simulink model "Throttle_harness"  (Simulink 7.7)
settings: Solver=FixedStepDiscrete  SolverMode=SingleTasking  StartTime=0.0  StopTime=100  FixedStep=.01  RelTol=1e-3
InitFcn:
  | if signalbuilder('Throttle_harness/Signal_Builder','activegroup') == 1
  |    CD_THROTTLE_PRIMARY_FUNCTION.DataType = 'uint8';
  |    CD_THROTTLE_PRIMARY_FUNCTION.Value = 255;
  | else
  |    CD_THROTTLE_PRIMARY_FUNCTION.DataType = 'uint8';
  |    CD_THROTTLE_PRIMARY_FUNCTION.Value = 0;
  | end
  | 
  | 
  | if signalbuilder('Throttle_harness/Signal_Builder','activegroup') == 3
  |    CD_THROTTLE_PRIMARY_DEBOUNCE_NORMAL.DataType = 'uint16';
  |    CD_THROTTLE_PRIMARY_DEBOUNCE_NORMAL.Value = 65535;
  | else
  |    CD_THROTTLE_PRIMARY_DEBOUNCE_NORMAL.DataType = 'uint16';
  |    CD_THROTTLE_PRIMARY_DEBOUNCE_NORMAL.Value = 10;
  | end
undefined symbols (not defined in the file): ACTIVE, CD_THROTTLE_FAULT_DERATE, CD_THROTTLE_PRI_RATIO_HIGH, CD_THROTTLE_PRI_RATIO_LOW, CD_THROTTLE_PRIMARY_DEBOUNCE_OORH, CD_THROTTLE_PRIMARY_DEBOUNCE_OORL, CD_THROTTLE_PRIMARY_FILTER_GAIN, CD_THROTTLE_PRIMARY_OORH, CD_THROTTLE_PRIMARY_OORL, INACTIVE, NON_FUNCTIONAL, NORMAL, OORH, OORL, sigbuilder_block, srate100, UNLIMITED
libraries: MX_Library x4, simulink x1
CloseFcn:
  | rtwprivate ssgencode ModelCloseRequest sle_main_controller
settings Model: Creator=spencermindeman  LastModifiedBy=aliebel  CovMetricSettings=dcmw  CovHTMLOptions=-aTS=1 -bRG=1 -bTC=1 -hTR=0 -nFC=0 -scm=1 -bcm=1 -xEv=0  covSaveCumulativeToWorkspaceVar=off  CovSaveSingleToWorkspaceVar=off  CovModelRefEnable=off
settings MATStruct: SampleTime=0.01  Offset=0  Priority=[1.0]
settings DataIOCC: LimitDataPoints=off  SaveOutput=off  SaveTime=off
settings OptimizationCC: BlockReduction=off  InlineParams=on  ExpressionFolding=off  StateBitsets=on  DataBitsets=on  UseTempVars=on  InitFltsAndDblsToZero=on  NoFixptDivByZeroProtection=on  EfficientFloat2IntCast=on  OptimizeModelRefInitCode=on
settings DebuggingCC: SaveWithParameterizedLinksMsg=none  MultiTaskDSMMsg=warning  MultiTaskCondExecSysMsg=none  IntegerOverflowMsg=none  ModelReferenceCSMismatchMessage=warning
settings HardwareCC: ProdBitPerInt=16  ProdBitPerPointer=16  ProdIntDivRoundTo=Floor  ProdEndianess=BigEndian  ProdWordSize=16  ProdHWDeviceType=Motorola HC12
settings ModelReferenceCC: ModelReferenceNumInstancesAllowed=Single
settings RTWCC: SystemTargetFile=ert.tlc  GenCodeOnly=on  TemplateMakefile=ert_default_tmf  Description=Real-Time Workshop Embedded Coder (no auto configuration)  GenerateReport=on  RetainRTWFile=on  ProcessScript=ert_make_rtw_hook  IncludeHyperlinkInReport=on  LaunchReport=on  IncludeERTFirstTime=on
settings RTWCC: CustomHeaderCode=|
  | #include "cpp_req_defines.h"
  | #include "hw_fin.h"
  | #include "cdata.h"
settings CodeAppCC: IgnoreCustomStorageClasses=off  DefineNamingRule=UpperCase
settings ERTTargetCC: TargetFcnLib=ansi_tfl_tmw.mat  FunctionExecutionProfile=off  MultiwordLength=2048  GenerateSampleERTMain=on  IncludeMdlTerminateFcn=off  SupportAbsoluteTime=off  SupportNonFinite=off  SupportComplex=off  PurelyIntegerCode=on  ERTCustomFileTemplate=gen_rtw_req_defines_h.tlc  GlobalDataDefinition=InSeparateSourceFile  GlobalDataReference=InSeparateHeaderFile  ConvertIfToSwitch=off

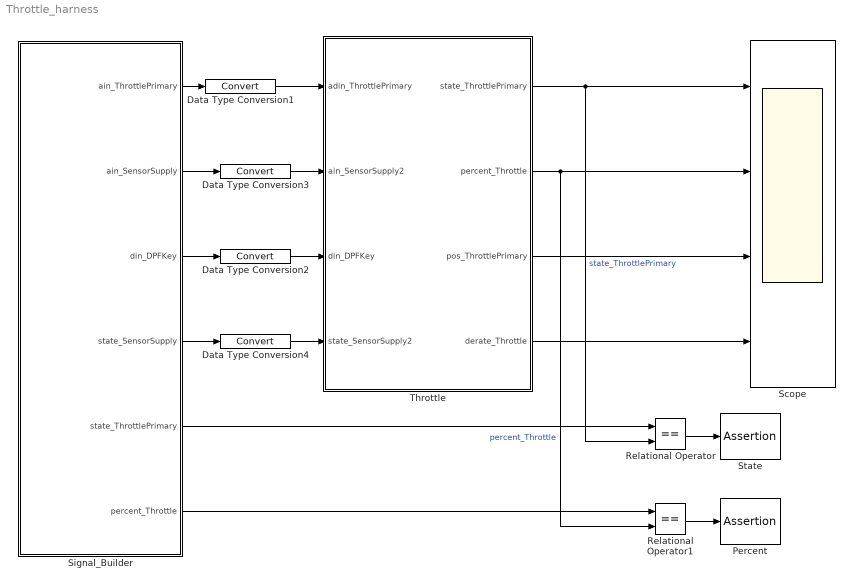
== system Throttle_harness ==
  Data Type Conversion{1..4} (4 alike) : DataTypeConversion
  Percent : Assertion  Enabled=off
  Relational Operator : RelationalOperator  Operator===  OutDataTypeStr=boolean
  Relational Operator1 : RelationalOperator  Operator===  OutDataTypeStr=boolean
  Scope : Scope  NumInputPorts=4
      settings: TimeRange=100  YMin=7.5~7.5~60~0  YMax=22.5~22.5~120~300  MaxDataPoints=50000
  Signal_Builder : Subsystem  Tag=STV Subsys  LoadFcn=sigbuilder_block('load');  StartFcn=sigbuilder_block('start');  StopFcn=sigbuilder_block('stop');  ClipboardFcn=sigbuilder_block('clipboard');  mask(Sigbuilder block){}
      mask help: Sigbuilder GUI
      mask init:
      | if ~strcmp(get_param(bdroot(gcbh),'SimulationStatus'),'stopped') tuvar = sigbuilder_block('maskInit'); end
      settings: CopyFcn=sigbuilder_block('copy');  DeleteFcn=sigbuilder_block('delete');  ModelCloseFcn=sigbuilder_block('modelClose');  PreSaveFcn=sigbuilder_block('preSave');  NameChangeFcn=sigbuilder_block('namechange');  OpenFcn=sigbuilder_block('open',[456.75 122.25 954 619.5 ]);  CloseFcn=sigbuilder_block('close');
      mask Display: plot(0,0,100,100,[10,10,40,40,10],[80,20,20,80,80],[40,10],[50,50], [40,27,10],[65,72,56],[40,25,25,10],[28,28,43,43]);
  State : Assertion  Enabled=off
  Throttle : Subsystem  TreatAsAtomicUnit=on  SystemSampleTime=srate100  RTWFileName=mod_Inputs
      settings: RTWSystemCode=Function  RTWFileNameOpts=User specified
  wires:
  Relational Operator/1 -> State/1
  Signal_Builder/1(ain_ThrottlePrimary) -> Data Type Conversion1/1
  Signal_Builder/3(din_DPFKey) -> Data Type Conversion2/1
  Data Type Conversion1/1 -> Throttle/1(adin_ThrottlePrimary)
  Data Type Conversion2/1 -> Throttle/3(din_DPFKey)
  Data Type Conversion3/1 -> Throttle/2(ain_SensorSupply2)
  Data Type Conversion4/1 -> Throttle/4(state_SensorSupply2)
  Throttle/1(state_ThrottlePrimary) -> Scope/1, Relational Operator/2  "state_ThrottlePrimary"
  Signal_Builder/2(ain_SensorSupply) -> Data Type Conversion3/1
  Signal_Builder/4(state_SensorSupply) -> Data Type Conversion4/1
  Signal_Builder/5(state_ThrottlePrimary) -> Relational Operator/1
  Relational Operator1/1 -> Percent/1
  Signal_Builder/6(percent_Throttle) -> Relational Operator1/1
  Throttle/2(percent_Throttle) -> Scope/2, Relational Operator1/2  "percent_Throttle"
  Throttle/3(pos_ThrottlePrimary) -> Scope/3
  Throttle/4(derate_Throttle) -> Scope/4

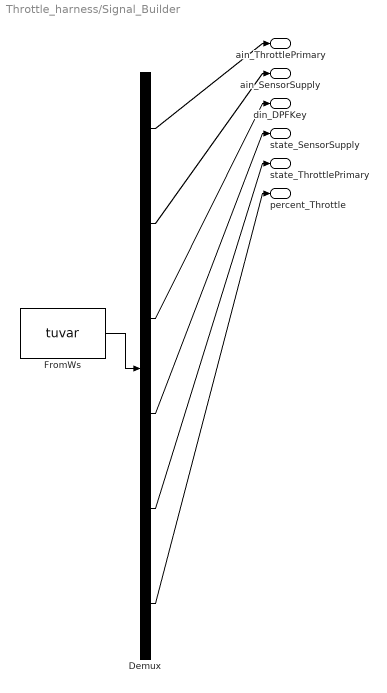
== system Throttle_harness/Signal_Builder ==
  Demux : Demux  Tag=STV Demux  Outputs=6
  FromWs : FromWorkspace  Tag=STV FromWs  VariableName=tuvar  SampleTime=0  SigBuilderData=DataTag0  VnvData=DataTag1
      SigBuilderData=|
      | common.afterFinalStr = 'Extrapolate'
      | common.sampleTime = 0
      | dataSet(1).timeRange = [0 100]
      | dataSet(1).name = 'T1-nonfunc'
      | dataSet(2).timeRange = [0 100]
      | dataSet(2).name = 'T2-OOR'
      | dataSet(3).timeRange = [0 100]
      | dataSet(3).name = 'T3-OOR_UNLIMITED'
      | dataSet(4).timeRange = [0 100]
      | dataSet(4).name = 'T4-Primary Only'
      | dataSet(5).timeRange = [0 100]
      | dataSet(5).name = 'T5-DPF Key'
      | sbobj.Groups(1).Name = 'T1-nonfunc'
      | sbobj.Groups(1).Signals(1).Name = 'ain_ThrottlePrimary'
      | sbobj.Groups(1).Signals(1).XData = [0 50 100]
      | sbobj.Groups(1).Signals(1).YData = [17 83 17]
      | sbobj.Groups(1).Signals(2).Name = 'ain_SensorSupply'
      | sbobj.Groups(1).Signals(2).XData = [0 100]
      | sbobj.Groups(1).Signals(2).YData = [500 500]
      | sbobj.Groups(1).Signals(3).Name = 'din_DPFKey'
      | sbobj.Groups(1).Signals(3).XData = [0 100]
      | sbobj.Groups(1).Signals(3).YData = [0 0]
      | sbobj.Groups(1).Signals(4).Name = 'state_SensorSupply'
      | sbobj.Groups(1).Signals(4).XData = [0 100]
      | sbobj.Groups(1).Signals(4).YData = [8 8]
      | sbobj.Groups(1).Signals(5).Name = 'state_ThrottlePrimary'
      | sbobj.Groups(1).Signals(5).XData = [0 100]
      | sbobj.Groups(1).Signals(5).YData = [8 8]
      | sbobj.Groups(1).Signals(6).Name = 'percent_Throttle'
      | sbobj.Groups(1).Signals(6).XData = [0 100]
      | sbobj.Groups(1).Signals(6).YData = [0 0]
      | sbobj.Groups(2).Name = 'T2-OOR'
      | sbobj.Groups(2).Signals(1).Name = 'ain_ThrottlePrimary'
      | sbobj.Groups(2).Signals(1).XData = [0 6.5 6.5 7.6 7.6 9.9 9.9 20 20 20.5 20.5 24.5 24.5 30 30 30.5 30.5 33.7 33.7 38.2 38.2 39.1 39.1 40 40 52.2 52.2 53.9 53.9 62.9 62.9 65.2 65.2 72 72 78 78 82.8 82.8 86.1 86.1 92.1 92.1 94.4 94.4 100]
      | sbobj.Groups(2).Signals(1).YData = [25 25 0 0 25 25 0 0 25 25 0 0 25 25 1023 1023 25 25 1023 1023 25 25 1023 1023 25 25 1023 1023 25 25 0 0 25 25 1023 1023 25 25 0 0 25 25 0 0 1023 1023]
      | sbobj.Groups(2).Signals(2).Name = 'ain_SensorSupply'
      | sbobj.Groups(2).Signals(2).XData = [0 100]
      | sbobj.Groups(2).Signals(2).YData = [500 500]
      | sbobj.Groups(2).Signals(3).Name = 'din_DPFKey'
      | sbobj.Groups(2).Signals(3).XData = [0 100]
      | sbobj.Groups(2).Signals(3).YData = [0 0]
      | sbobj.Groups(2).Signals(4).Name = 'state_SensorSupply'
      | sbobj.Groups(2).Signals(4).XData = [0 52.2 52.2 54.4 54.4 61.6 61.6 65.4 65.4 73.2 73.2 80.1 80.1 84.8 84.8 89.6 89.6 100]
      | sbobj.Groups(2).Signals(4).YData = [8 8 22 22 8 8 21 21 8 8 22 22 8 8 21 21 8 8]
      | sbobj.Groups(2).Signals(5).Name = 'state_ThrottlePrimary'
      | sbobj.Groups(2).Signals(5).XData = [0 11.8 11.8 25.8 25.8 35.2 35.2 41.5 41.5 84.8 84.8 87.4 87.4 94 94 95.9 95.9 100]
      | sbobj.Groups(2).Signals(5).YData = [8 8 22 22 8 8 21 21 8 8 22 22 8 8 22 22 21 21]
      | sbobj.Groups(2).Signals(6).Name = 'percent_Throttle'
      | sbobj.Groups(2).Signals(6).XData = [0 0.1 0.1 11.8 11.8 25.9 25.9 35.2 35.2 41.6 41.6 52.2 52.2 54.6 54.6 61.6 61.6 65.5 65.5 73.2 73.2 80.2 80.2 84.8 84.8 89.7 89.7 94 94 100]
      | sbobj.Groups(2).Signals(6).YData = [0 0 46 46 500 500 46 46 500 500 46 46 500 500 46 46 500 500 46 46 500 500 46 46 500 500 46 46 500 500]
      | sbobj.Groups(3).Name = 'T3-OOR_UNLIMITED'
      | sbobj.Groups(3).Signals(1).Name = 'ain_ThrottlePrimary'
      | sbobj.Groups(3).Signals(1).XData = [0 6.5 6.5 7.6 7.6 9.9 9.9 20 20 20.5 20.5 24.5 24.5 30 30 30.5 30.5 33.7 33.7 38.2 38.2 39.1 39.1 40 40 100]
      | sbobj.Groups(3).Signals(1).YData = [25 25 0 0 25 25 0 0 25 25 0 0 25 25 1023 1023 25 25 1023 1023 25 25 1023 1023 25 25]
      | sbobj.Groups(3).Signals(2).Name = 'ain_SensorSupply'
      | sbobj.Groups(3).Signals(2).XData = [0 100]
      | sbobj.Groups(3).Signals(2).YData = [500 500]
      | sbobj.Groups(3).Signals(3).Name = 'din_DPFKey'
      | sbobj.Groups(3).Signals(3).XData = [0 100]
      | sbobj.Groups(3).Signals(3).YData = [0 0]
      | sbobj.Groups(3).Signals(4).Name = 'state_SensorSupply'
      | sbobj.Groups(3).Signals(4).XData = [0 100]
      | sbobj.Groups(3).Signals(4).YData = [8 8]
      | sbobj.Groups(3).Signals(5).Name = 'state_ThrottlePrimary'
      | sbobj.Groups(3).Signals(5).XData = [0 11.8 11.8 35.2 35.2 100]
      | sbobj.Groups(3).Signals(5).YData = [8 8 22 22 21 21]
      | sbobj.Groups(3).Signals(6).Name = 'percent_Throttle'
      | sbobj.Groups(3).Signals(6).XData = [0 0.1 0.1 11.8 11.8 100]
      | sbobj.Groups(3).Signals(6).YData = [0 0 46 46 500 500]
      | sbobj.Groups(4).Name = 'T4-Primary Only'
      | sbobj.Groups(4).Signals(1).Name = 'ain_ThrottlePrimary'
      | sbobj.Groups(4).Signals(1).XData = [0 30 30 40 40 100]
      | sbobj.Groups(4).Signals(1).YData = [25 25 0 0 25 25]
      | sbobj.Groups(4).Signals(2).Name = 'ain_SensorSupply'
      | sbobj.Groups(4).Signals(2).XData = [0 100]
      | sbobj.Groups(4).Signals(2).YData = [500 500]
      | sbobj.Groups(4).Signals(3).Name = 'din_DPFKey'
      | sbobj.Groups(4).Signals(3).XData = [0 100]
      | sbobj.Groups(4).Signals(3).YData = [0 0]
      | sbobj.Groups(4).Signals(4).Name = 'state_SensorSupply'
      | sbobj.Groups(4).Signals(4).XData = [0 10 10 20 20 100]
      | sbobj.Groups(4).Signals(4).YData = [8 8 21 21 8 8]
      | sbobj.Groups(4).Signals(5).Name = 'state_ThrottlePrimary'
      | sbobj.Groups(4).Signals(5).XData = [0 31.9 31.9 41.3 41.3 100]
      | sbobj.Groups(4).Signals(5).YData = [8 8 22 22 8 8]
      | sbobj.Groups(4).Signals(6).Name = 'percent_Throttle'
      | sbobj.Groups(4).Signals(6).XData = [0 0.1 0.1 10 10 20.1 20.1 31.9 31.9 41.4 41.4 100]
      | sbobj.Groups(4).Signals(6).YData = [0 0 46 46 500 500 46 46 500 500 46 46]
      | sbobj.Groups(5).Name = 'T5-DPF Key'
      | sbobj.Groups(5).Signals(1).Name = 'ain_ThrottlePrimary'
      | sbobj.Groups(5).Signals(1).XData = [0 20 30 59.9 74.8 100]
      | sbobj.Groups(5).Signals(1).YData = [25 25 25 25 25 25]
      | sbobj.Groups(5).Signals(2).Name = 'ain_SensorSupply'
      | sbobj.Groups(5).Signals(2).XData = [0 100]
      | sbobj.Groups(5).Signals(2).YData = [500 500]
      | sbobj.Groups(5).Signals(3).Name = 'din_DPFKey'
      | sbobj.Groups(5).Signals(3).XData = [0 5.4 5.4 7.2 7.2 18.8 18.8 20.3 20.3 100]
      | sbobj.Groups(5).Signals(3).YData = [0 0 1 1 0 0 1 1 0 0]
      | sbobj.Groups(5).Signals(4).Name = 'state_SensorSupply'
      | sbobj.Groups(5).Signals(4).XData = [0 17.4 17.4 21.4 21.4 100]
      | sbobj.Groups(5).Signals(4).YData = [8 8 21 21 8 8]
      | sbobj.Groups(5).Signals(5).Name = 'state_ThrottlePrimary'
      | sbobj.Groups(5).Signals(5).XData = [0 100]
      | sbobj.Groups(5).Signals(5).YData = [8 8]
      | sbobj.Groups(5).Signals(6).Name = 'percent_Throttle'
      | sbobj.Groups(5).Signals(6).XData = [0 0.1 0.1 5.4 5.4 7.3 7.3 17.4 17.4 18.8 18.8 20.4 20.4 21.5 21.5 100]
      | sbobj.Groups(5).Signals(6).YData = [0 0 46 46 0 0 46 46 500 500 0 0 500 500 46 46]
  ain_ThrottlePrimary : Outport  Tag=STV Outport
  ain_SensorSupply : Outport  Tag=STV Outport  Port=2
  din_DPFKey : Outport  Tag=STV Outport  Port=3
  state_SensorSupply : Outport  Tag=STV Outport  Port=4
  state_ThrottlePrimary : Outport  Tag=STV Outport  Port=5
  percent_Throttle : Outport  Tag=STV Outport  Port=6
  wires:
  FromWs/1 -> Demux/1
  Demux/1 -> ain_ThrottlePrimary/1
  Demux/2 -> ain_SensorSupply/1
  Demux/3 -> din_DPFKey/1
  Demux/4 -> state_SensorSupply/1
  Demux/5 -> state_ThrottlePrimary/1
  Demux/6 -> percent_Throttle/1

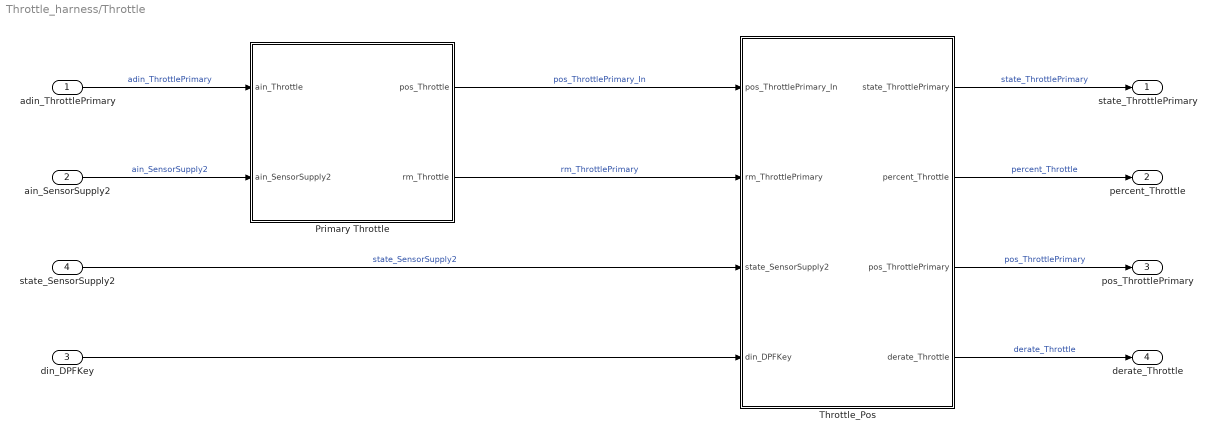
== system Throttle_harness/Throttle ==
  adin_ThrottlePrimary : Inport  OutDataTypeStr=uint16
  ain_SensorSupply2 : Inport  Port=2  OutDataTypeStr=uint16
  din_DPFKey : Inport  Port=3
  state_SensorSupply2 : Inport  Port=4  OutDataTypeStr=uint8
  Primary Throttle : Subsystem
  Throttle_Pos : Stateflow chart  TreatAsAtomicUnit=on
  state_ThrottlePrimary : Outport
  percent_Throttle : Outport  Port=2
  pos_ThrottlePrimary : Outport  Port=3
  derate_Throttle : Outport  Port=4
  wires:
  adin_ThrottlePrimary/1 -> Primary Throttle/1(ain_Throttle)  "adin_ThrottlePrimary"
  Throttle_Pos/1(state_ThrottlePrimary) -> state_ThrottlePrimary/1  "state_ThrottlePrimary"
  ain_SensorSupply2/1 -> Primary Throttle/2(ain_SensorSupply2)  "ain_SensorSupply2"
  Throttle_Pos/2(percent_Throttle) -> percent_Throttle/1  "percent_Throttle"
  Primary Throttle/1(pos_Throttle) -> Throttle_Pos/1(pos_ThrottlePrimary_In)  "pos_ThrottlePrimary_In"
  Primary Throttle/2(rm_Throttle) -> Throttle_Pos/2(rm_ThrottlePrimary)  "rm_ThrottlePrimary"
  Throttle_Pos/3(pos_ThrottlePrimary) -> pos_ThrottlePrimary/1  "pos_ThrottlePrimary"
  state_SensorSupply2/1 -> Throttle_Pos/3(state_SensorSupply2)  "state_SensorSupply2"
  Throttle_Pos/4(derate_Throttle) -> derate_Throttle/1  "derate_Throttle"
  din_DPFKey/1 -> Throttle_Pos/4(din_DPFKey)

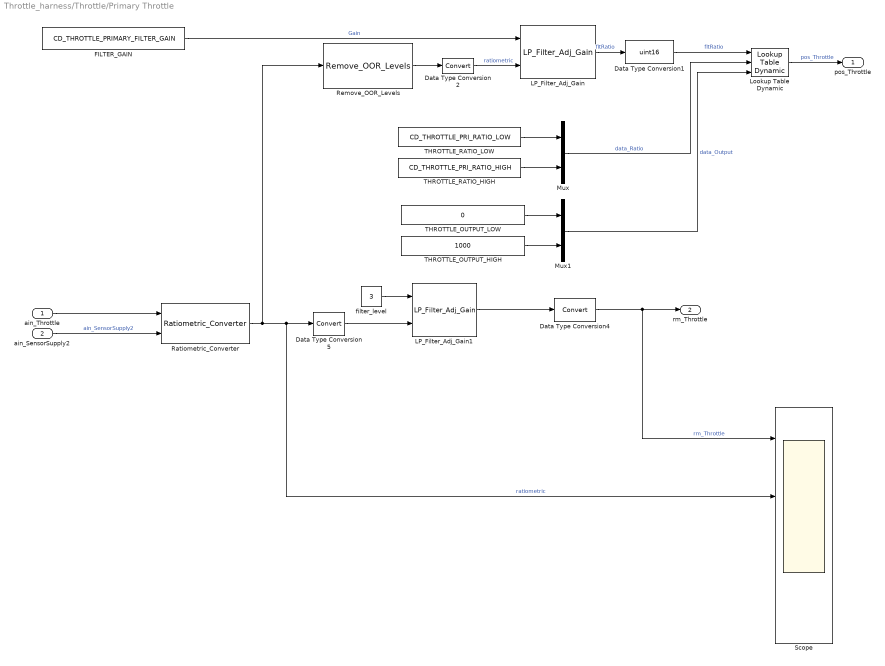
== system Throttle_harness/Throttle/Primary Throttle ==
  ain_Throttle : Inport
  ain_SensorSupply2 : Inport  Port=2
  Data Type Conversion1 : DataTypeConversion  OutDataTypeStr=uint16
  Data Type Conversion2 : DataTypeConversion
  Data Type Conversion4 : DataTypeConversion
  Data Type Conversion5 : DataTypeConversion
  FILTER_GAIN : Constant  Value=CD_THROTTLE_PRIMARY_FILTER_GAIN  OutDataTypeStr=uint8  SampleTime=-1
  LP_Filter_Adj_Gain : MX_Library/LP_Filter_Adj_Gain  SystemSampleTime=-1
  LP_Filter_Adj_Gain1 : MX_Library/LP_Filter_Adj_Gain  SystemSampleTime=-1
  Lookup Table Dynamic : simulink/Lookup Tables/Lookup Table Dynamic  LookUpMeth=Interpolation-Use End Values  OutDataTypeStr=fixdt(0,16,0)  OutputDataTypeScalingMode=Specify via dialog  OutDataType=fixdt(0,16,0)  OutScaling=[]  DoSatur=off
  Mux : Mux  Inputs=2
  Mux1 : Mux  Inputs=2
  Ratiometric_Converter : MX_Library/Ratiometric_Converter  SystemSampleTime=-1  multiplier=CD_THROTTLE_PRIMARY_RATIO_MULTIPLIER
  Remove_OOR_Levels : MX_Library/Remove_OOR_Levels  SystemSampleTime=-1  OORL_LEVEL=50  OORH_LEVEL=950
  Scope : Scope  NumInputPorts=4
      settings: TimeRange=100  YMin=7.5~7.5~60~0  YMax=22.5~22.5~120~300  MaxDataPoints=50000
  THROTTLE_OUTPUT_HIGH : Constant  Value=1000  OutDataTypeStr=uint16  SampleTime=-1
  THROTTLE_OUTPUT_LOW : Constant  Value=0  OutDataTypeStr=uint16  SampleTime=-1
  THROTTLE_RATIO_HIGH : Constant  Value=CD_THROTTLE_PRI_RATIO_HIGH  OutDataTypeStr=uint16  SampleTime=-1
  THROTTLE_RATIO_LOW : Constant  Value=CD_THROTTLE_PRI_RATIO_LOW  OutDataTypeStr=uint16  SampleTime=-1
  filter_level : Constant  Value=3  OutDataTypeStr=uint8  SampleTime=-1
  pos_Throttle : Outport
  rm_Throttle : Outport  Port=2
  wires:
  Data Type Conversion5/1 -> LP_Filter_Adj_Gain1/2
  filter_level/1 -> LP_Filter_Adj_Gain1/1
  LP_Filter_Adj_Gain1/1 -> Data Type Conversion4/1
  Data Type Conversion2/1 -> LP_Filter_Adj_Gain/2  "ratiometric"
  Remove_OOR_Levels/1 -> Data Type Conversion2/1
  Data Type Conversion4/1 -> rm_Throttle/1, Scope/1  "rm_Throttle"
  Ratiometric_Converter/1 -> Remove_OOR_Levels/1, Data Type Conversion5/1, Scope/2  "ratiometric"
  FILTER_GAIN/1 -> LP_Filter_Adj_Gain/1  "Gain"
  Data Type Conversion1/1 -> Lookup Table Dynamic/1  "fltRatio"
  LP_Filter_Adj_Gain/1 -> Data Type Conversion1/1  "fltRatio"
  ain_SensorSupply2/1 -> Ratiometric_Converter/2  "ain_SensorSupply2"
  ain_Throttle/1 -> Ratiometric_Converter/1
  Lookup Table Dynamic/1 -> pos_Throttle/1  "pos_Throttle"
  THROTTLE_RATIO_LOW/1 -> Mux/1
  THROTTLE_OUTPUT_HIGH/1 -> Mux1/2
  Mux/1 -> Lookup Table Dynamic/2  "data_Ratio"
  THROTTLE_OUTPUT_LOW/1 -> Mux1/1
  Mux1/1 -> Lookup Table Dynamic/3  "data_Output"
  THROTTLE_RATIO_HIGH/1 -> Mux/2

== stateflow chart Throttle/Throttle_Pos ==
  state THROTTLE_POSITION [parallel]
    settings: executionOrder=2
    state PARKED_REGEN
      en: percent_Throttle = 0;
    state NORMAL
      state NO_THROTTLE
        en:percent_Throttle = CD_THROTTLE_FAULT_DERATE * 10;  // Value is percent (0 to 1000), mulitply by 10 to get correct resolution
        en:derate_Throttle = CD_THROTTLE_FAULT_DERATE;
      state VALID
        du:percent_Throttle = pos_ThrottlePrimary;
        en:derate_Throttle = 0;
      (default) -> VALID
      NO_THROTTLE -> VALID : [(state_ThrottlePrimary == NORMAL)...
          | && (state_SensorSupply2 == NORMAL)]
      VALID -> NO_THROTTLE : [(state_ThrottlePrimary != NORMAL)...
          | || (state_SensorSupply2 != NORMAL)]
    PARKED_REGEN -> THROTTLE_POSITION.NORMAL : [(din_DPFKey == INACTIVE)]
    THROTTLE_POSITION.NORMAL -> PARKED_REGEN : [(din_DPFKey == ACTIVE)]
    (default) -> THROTTLE_POSITION.NORMAL
  state THROTTLE_PRIMARY [parallel]
    settings: executionOrder=1
    state NON_FUNCTIONAL
      en:state_ThrottlePrimary = NORMAL;
      en:pos_ThrottlePrimary = 0;
    state NORMAL
      en:state_ThrottlePrimary = NORMAL;
      en:pos_ThrottlePrimary = pos_ThrottlePrimary_In;
      du:pos_ThrottlePrimary = pos_ThrottlePrimary_In;
    state OORH
      state NORMAL
        en:state_ThrottlePrimary = OORH;
        en:pos_ThrottlePrimary = 0;
      state DEBOUNCE
        en:debouncePrimary = 0;
        du:debouncePrimary++;
      THROTTLE_PRIMARY.OORH.DEBOUNCE -> THROTTLE_PRIMARY.OORH.NORMAL : [(debouncePrimary >= CD_THROTTLE_PRIMARY_DEBOUNCE_OORH)...
          | || (state_ThrottlePrimary == OORH)]
      (default) -> THROTTLE_PRIMARY.OORH.DEBOUNCE
    state OORL
      state NORMAL
        en:state_ThrottlePrimary = OORL;
        en:pos_ThrottlePrimary = 0;
      state DEBOUNCE
        en:debouncePrimary = 0;
        du:debouncePrimary++;
      (default) -> THROTTLE_PRIMARY.OORL.DEBOUNCE
      THROTTLE_PRIMARY.OORL.DEBOUNCE -> THROTTLE_PRIMARY.OORL.NORMAL : [(debouncePrimary >= CD_THROTTLE_PRIMARY_DEBOUNCE_OORL)...
          | || (state_ThrottlePrimary == OORL)]
    state DEBOUNCE_NORMAL
      state NORMAL
        en:state_ThrottlePrimary = NORMAL;
      state DEBOUNCE
        en:debouncePrimary = 0;
        du:debouncePrimary++;
      (default) -> THROTTLE_PRIMARY.DEBOUNCE_NORMAL.DEBOUNCE
      THROTTLE_PRIMARY.DEBOUNCE_NORMAL.DEBOUNCE -> THROTTLE_PRIMARY.DEBOUNCE_NORMAL.NORMAL : [((CD_THROTTLE_PRIMARY_DEBOUNCE_NORMAL != UNLIMITED)...
          | && (debouncePrimary >= CD_THROTTLE_PRIMARY_DEBOUNCE_NORMAL))]
    OORL -> DEBOUNCE_NORMAL : [(rm_ThrottlePrimary > CD_THROTTLE_PRIMARY_OORL)...
        | || (state_SensorSupply2 != NORMAL)]
    OORH -> DEBOUNCE_NORMAL : [(rm_ThrottlePrimary < CD_THROTTLE_PRIMARY_OORH)...
        | || (state_SensorSupply2 != NORMAL)]
    THROTTLE_PRIMARY.NORMAL -> OORH [order 1] : [(rm_ThrottlePrimary >= CD_THROTTLE_PRIMARY_OORH)...
        | && (state_SensorSupply2 == NORMAL)]
    (default) -> NON_FUNCTIONAL
    THROTTLE_PRIMARY.NORMAL -> OORL [order 2] : [(rm_ThrottlePrimary <= CD_THROTTLE_PRIMARY_OORL)...
        | && (state_SensorSupply2 == NORMAL)]
    NON_FUNCTIONAL -> THROTTLE_PRIMARY.NORMAL : [(CD_THROTTLE_PRIMARY_FUNCTION != NON_FUNCTIONAL)]
    DEBOUNCE_NORMAL -> THROTTLE_PRIMARY.NORMAL [order 1] : [(state_ThrottlePrimary == NORMAL)]
    DEBOUNCE_NORMAL -> OORL [order 3] : [(rm_ThrottlePrimary <= CD_THROTTLE_PRIMARY_OORL)]
    DEBOUNCE_NORMAL -> OORH [order 2] : [(rm_ThrottlePrimary >= CD_THROTTLE_PRIMARY_OORH)]
  data: pos_ThrottlePrimary_In input uint16; rm_ThrottlePrimary input uint16; state_ThrottlePrimary output uint8; debouncePrimary local uint16 =0; OORH parameter uint8 =21; OORL parameter uint8 =22; NON_FUNCTIONAL parameter uint8 =255; NORMAL parameter uint8 =8; percent_Throttle output uint16; CD_THROTTLE_PRIMARY_FUNCTION parameter uint8; CD_THROTTLE_PRIMARY_OORL parameter uint16; CD_THROTTLE_PRIMARY_OORH parameter uint16; CD_THROTTLE_PRIMARY_DEBOUNCE_OORL parameter uint16; pos_ThrottlePrimary output uint16; state_SensorSupply2 input uint8; CD_THROTTLE_PRIMARY_DEBOUNCE_OORH parameter uint16; CD_THROTTLE_PRIMARY_DEBOUNCE_NORMAL parameter uint16; UNLIMITED parameter uint16; derate_Throttle output uint8; CD_THROTTLE_FAULT_DERATE parameter uint8; din_DPFKey input boolean; ACTIVE parameter uint8; INACTIVE parameter uint8
